simulink model "rc_value_calc"  (R2013a)
settings: Solver=ode45  StartTime=0.0  StopTime=10.0  RelTol=1e-3
settings Model: Creator=hlopez5  LastModifiedBy=hlopez5

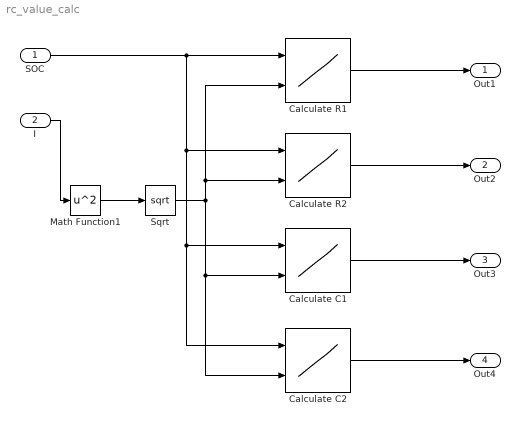
== system rc_value_calc ==
  "SOC " : Inport
  I : Inport  Port=2
  Calculate C1 : Lookup_n-D  BreakpointsForDimension1=[1:3]  BreakpointsForDimension2=[1:3]  RndMeth=Simplest  InputSameDT=on
  Calculate C2 : Lookup_n-D  BreakpointsForDimension1=[1:3]  BreakpointsForDimension2=[1:3]  RndMeth=Simplest  InputSameDT=on
  Calculate R1 : Lookup_n-D  BreakpointsForDimension1=[1:3]  BreakpointsForDimension2=[1:3]  RndMeth=Simplest  InputSameDT=on
  Calculate R2 : Lookup_n-D  BreakpointsForDimension1=[1:3]  BreakpointsForDimension2=[1:3]  RndMeth=Simplest  InputSameDT=on
  Math Function1 : Math  Operator=square  SaturateOnIntegerOverflow=on
  Sqrt : Sqrt  SaturateOnIntegerOverflow=on
  Out1 : Outport
  Out2 : Outport  Port=2
  Out3 : Outport  Port=3
  Out4 : Outport  Port=4
  wires:
  I/1 -> Math Function1/1
  Math Function1/1 -> Sqrt/1
  Calculate R1/1 -> Out1/1
  Calculate R2/1 -> Out2/1
  Calculate C1/1 -> Out3/1
  Calculate C2/1 -> Out4/1
  Sqrt/1 -> Calculate R2/2, Calculate R1/2, Calculate C2/2, Calculate C1/2
  "SOC "/1 -> Calculate C2/1, Calculate C1/1, Calculate R2/1, Calculate R1/1
